simulink model "DC_Link"  (R2020b)
settings: Solver=VariableStepAuto  StartTime=0.0  StopTime=2/80e3  RelTol=1e-3
InitFcn:
  | SampleTime=1e-7;
  | P_IPT=40;
  | I_tx=5;
  | Im=5;
libraries: powerlib x1
settings Model: Creator=enes_  LastModifiedBy=enes_
settings DataIOCC: ReturnWorkspaceOutputs=off

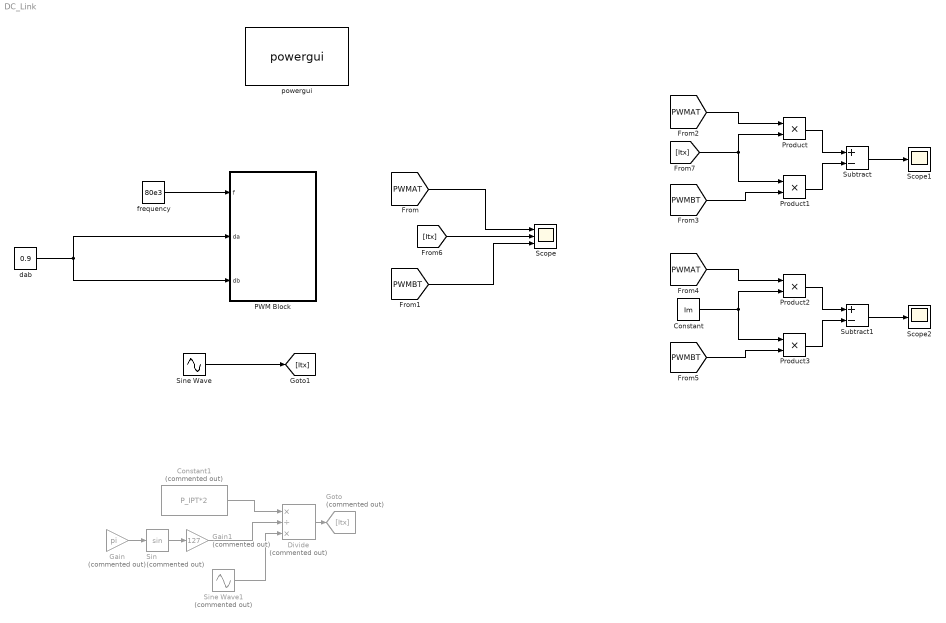
== system DC_Link ==
  Constant : Constant  Value=Im
  Constant1 : Constant  Commented=on  Value=P_IPT*2
  Divide : Product  Commented=on  Inputs=*/*
  Gain : Gain  Commented=on  Gain=pi
  Gain1 : Gain  Commented=on  Gain=127
  Goto : Goto  Commented=on  GotoTag=Itx
  PWM Block : Subsystem
  Product{,1..3} (4 alike) : Product
  Scope : Scope  NumInputPorts=3
  Scope1 : Scope
  Scope2 : Scope
  Sin : Trigonometry  Commented=on
  Sine Wave : Sin  Amplitude=I_tx  Frequency=80e3*2*pi  Phase=pi  SampleTime=SampleTime
  Sine Wave1 : Sin  Commented=on  Frequency=80e3*2*pi  Phase=pi  SampleTime=SampleTime
  Subtract : Sum  Inputs=+-
  Subtract1 : Sum  Inputs=+-
  dab : Constant  Value=0.9
  frequency : Constant  Value=80e3
  powergui : powerlib/powergui  Priority=1  SimulationMode=Discrete  SampleTime=SampleTime  frequency=60  Iterations=50  frequencyindice=0  Pbase=100e6  ErrMax=1e-4  UnitsV=kV  UnitsW=MW  buscounter=0  FunctionMessages=off  echomessages=off  EnableUseOfTLC=off  CurrentSourceSwitches=off  DisableSnubberDevices=off  DisableRonSwitches=off  DisableVfSwitches=off  DisplayEquations=off  AutomaticDiscreteSolvers=off  SolverType=Tustin/Backward Euler (TBE)  Interpol=off  ExternalGateDelay=off  methode=off  Ts=100  x0status=blocks  SPID=on  SwTol=0  HookPort=off  NonlinearTolerance=1e-4  nMaxIteration=100  ContinueOnMaxIteration=off  RestoreLinks=warning  ResistiveCurrentMeasurement=off  Frange=[1e3:1e3:240e3]  Ylog=off  Xlog=on  ShowGrid=off  save=off  variable=ZData  structure=Itx_cap  ZoomFFT=off  StartTime=0.0  cycles=1  DisplayStyle=2  fundamental=80000  FreqAxis=on  MaxFrequency=9*80000  frequencyindicesteady=1  RmsSteady=1  display=off
  wires:
  frequency/1 -> PWM Block/1(f)
  [PWMAT] -> Scope/1
  [Itx] -> Scope/2
  [PWMBT] -> Scope/3
  [PWMAT] -> Product/1
  [Itx] -> Product/2, Product1/1
  [PWMBT] -> Product1/2
  Product/1 -> Subtract/1
  Product1/1 -> Subtract/2
  Subtract/1 -> Scope1/1
  Constant/1 -> Product2/2, Product3/1
  [PWMBT] -> Product3/2
  Subtract1/1 -> Scope2/1
  Product3/1 -> Subtract1/2
  Product2/1 -> Subtract1/1
  [PWMAT] -> Product2/1
  Gain/1 -> Sin/1
  Constant1/1 -> Divide/1
  Sine Wave1/1 -> Divide/3
  Divide/1 -> Goto/1
  Gain1/1 -> Divide/2
  Sin/1 -> Gain1/1
  dab/1 -> PWM Block/2(da), PWM Block/3(db)
  Sine Wave/1 -> [Itx]

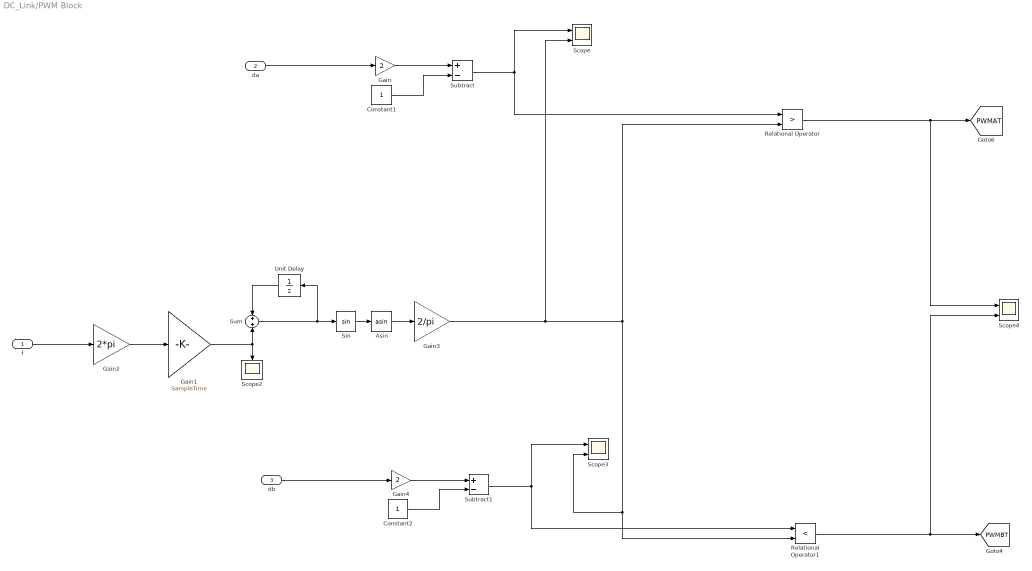
== system DC_Link/PWM Block ==
  f : Inport
  da : Inport  Port=2
  db : Inport  Port=3
  Asin : Trigonometry  Operator=asin
  Constant1 : Constant
  Constant2 : Constant
  Gain : Gain  Gain=2
  Gain1 : Gain  Gain=SampleTime
  Gain2 : Gain  Gain=2*pi
  Gain3 : Gain  Gain=2/pi
  Gain4 : Gain  Gain=2
  Relational Operator : RelationalOperator  Operator=>  OutDataTypeStr=boolean  RndMeth=Simplest
  Relational Operator1 : RelationalOperator  Operator=<  OutDataTypeStr=boolean  RndMeth=Simplest
  Scope : Scope  NumInputPorts=2
  Scope2 : Scope
  Scope3 : Scope  NumInputPorts=2
  Scope4 : Scope  NumInputPorts=2
  Sin : Trigonometry
  Subtract : Sum  Inputs=+-
  Subtract1 : Sum  Inputs=+-
  Sum : Sum
  Unit Delay : UnitDelay  SampleTime=-1  HasFrameUpgradeWarning=on
  tag scope: PWMAT=global, PWMBT=global
  wires:
  da/1 -> Gain/1
  Gain/1 -> Subtract/1
  Constant1/1 -> Subtract/2
  Subtract/1 -> Scope/1, Relational Operator/1
  Sin/1 -> Asin/1
  Asin/1 -> Gain3/1
  Sum/1 -> Sin/1, Unit Delay/1
  Unit Delay/1 -> Sum/1
  Gain2/1 -> Gain1/1
  Gain1/1 -> Sum/2, Scope2/1
  f/1 -> Gain2/1
  Gain3/1 -> Scope/2, Scope3/2, Relational Operator1/2, Relational Operator/2
  Gain4/1 -> Subtract1/1
  Relational Operator1/1 -> [PWMBT], Scope4/2
  db/1 -> Gain4/1
  Constant2/1 -> Subtract1/2
  Subtract1/1 -> Scope3/1, Relational Operator1/1
  Relational Operator/1 -> Scope4/1, [PWMAT]
